simulink model "mdl5"  (R2014a)
settings: Solver=FixedStepDiscrete  SolverMode=SingleTasking  StartTime=TIME(1)  StopTime=TIME(end)  FixedStep=SIMSTEP  RelTol=1e-3
model workspace (MAT data in the model file):
  autoc_mdd_data01 : struct (value not decoded)
values from neighbouring files (symbols this model uses):
  map_mr4_01 = [400 500 600 700 800 900 1000 1100 1200 1300 1400 1500 ... (47 elements, 1x47)]    [scr_simdata_all.mat]
  map_mr4_02 = [0.684 0.622 0.566 0.514 0.468 0.425 0.387 0.352 0.32 0.291 0.264 0.241 ... (47 elements, 1x47)]    [scr_simdata_all.mat]
  map_mr4_03 = [10 12 14 16 18 20 22 24 26 28 30 32 ... (51 elements, 1x51)]    [scr_simdata_all.mat]
  map_mr4_04 = [0.0257 0.0124 0.00595 0.00286 0.00137 0.000662 0.000318 0.000153 7.37e-05 3.54e-05 1.7e-05 8.19e-06 ... (51 elements, 1x51)]    [scr_simdata_all.mat]
  map_mr4_05 = [10 12 14 16 18 20 22 24 26 28 30 32 ... (51 elements, 1x51)]    [scr_simdata_all.mat]
  map_mr4_06 = [0.9647 0.9835 0.9945 0.9994 0.9972 0.9871 0.97 0.9462 0.9163 0.8807 0.8403 0.796 ... (51 elements, 1x51)]    [scr_simdata_all.mat]
  map_mr4_07 = [0 1 2 3 4 5 6 7 8 9 10 11 ... (51 elements, 1x51)]    [scr_simdata_all.mat]
  map_mr4_08 = [0 0.01 0.0214 0.0335 0.0459 0.0587 0.0718 0.085 0.0985 0.112 0.126 0.14 ... (51 elements, 1x51)]    [scr_simdata_all.mat]
  Parameter114 = 126    [scr_simdata_all.mat]
  Parameter115 = 129    [scr_simdata_all.mat]
  Parameter131 = 3    [scr_simdata_all.mat]
  Parameter141 = 0    [scr_simdata_all.mat]
  Parameter143 = 1    [scr_simdata_all.mat]
  Parameter144 = 3    [scr_simdata_all.mat]
  Parameter51 = 0    [scr_simdata_all.mat]
  Parameter52 = 1    [scr_simdata_all.mat]
  Parameter53 = 2    [scr_simdata_all.mat]
  Parameter70 = 30    [scr_simdata_all.mat]
  Parameter71 = 33    [scr_simdata_all.mat]
  Parameter92 = 78    [scr_simdata_all.mat]
  Parameter93 = 81    [scr_simdata_all.mat]
  SIMSTEP = 0.0001024    [scr_simdata_all.mat]
(part 4 of 4)

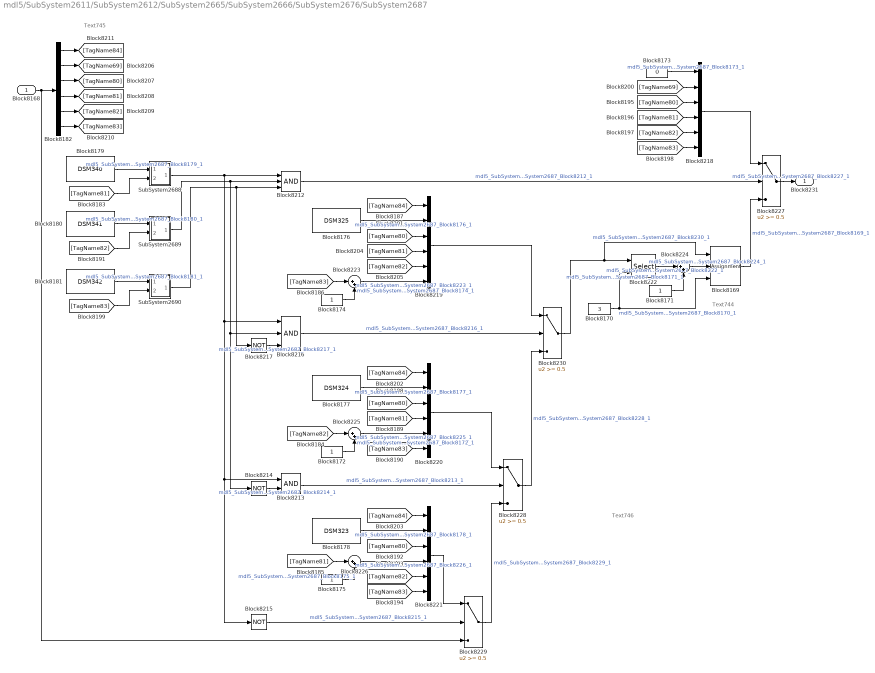
== system mdl5/SubSystem2611/SubSystem2612/SubSystem2665/SubSystem2666/SubSystem2676/SubSystem2687 ==
  note: Text746
  note: Text745
  note: Text744
  Block8168 : Inport
  Block8169 : Assignment  IndexOptions=Index vector (port)  OutputSizes=[1 1]
  Block8170 : Constant  Value=3  OutDataTypeStr=double  SampleTime=-1
  Block{8171..8172,8174..8175} (4 alike) : Constant  OutDataTypeStr=double  SampleTime=-1
  Block8173 : Constant  Value=0  OutDataTypeStr=double  SampleTime=-1
  Block8176 : DataStoreRead  DataStoreName=DSM325
  Block8177 : DataStoreRead  DataStoreName=DSM324
  Block8178 : DataStoreRead  DataStoreName=DSM323
  Block8179 : DataStoreRead  DataStoreName=DSM340
  Block8180 : DataStoreRead  DataStoreName=DSM341
  Block8181 : DataStoreRead  DataStoreName=DSM342
  Block8182 : Demux  Outputs=6
  Block8212 : Logic  Inputs=3
  Block8213 : Logic
  Block8214 : Logic  Operator=NOT
  Block8215 : Logic  Operator=NOT
  Block8216 : Logic  Inputs=3
  Block8217 : Logic  Operator=NOT
  Block{8218..8221} (4 alike) : Mux  Inputs=6
  Block8222 : Selector  IndexOptions=Index vector (port)  Indices=[1 3]
  Block{8223..8226} (4 alike) : Sum  Inputs=|++  OutDataTypeStr=double  RndMeth=Zero  SaturateOnIntegerOverflow=on  InputSameDT=on
  Block{8227..8230} (4 alike) : Switch  Threshold=0.5  RndMeth=Zero  SaturateOnIntegerOverflow=on  InputSameDT=on
  SubSystem2688 : Subsystem
  SubSystem2689 : Subsystem
  SubSystem2690 : Subsystem
  Block8231 : Outport
  wires:
  SubSystem2688/1(Out1) -> Block8212/1, Block8216/1, Block8213/1, Block8215/1
  SubSystem2689/1(Out1) -> Block8212/2, Block8216/2, Block8214/1
  SubSystem2690/1(Out1) -> Block8212/3, Block8217/1
  Block8212/1 -> Block8227/2  "mdl5_SubSystem2611_SubSystem2612_SubSystem2665_SubSystem2666_SubSystem2676_SubSystem2687_Block8212_1"
  Block8213/1 -> Block8228/2  "mdl5_SubSystem2611_SubSystem2612_SubSystem2665_SubSystem2666_SubSystem2676_SubSystem2687_Block8213_1"
  Block8215/1 -> Block8229/2  "mdl5_SubSystem2611_SubSystem2612_SubSystem2665_SubSystem2666_SubSystem2676_SubSystem2687_Block8215_1"
  Block8218/1 -> Block8227/1
  Block8179/1 -> SubSystem2688/1(In1)  "mdl5_SubSystem2611_SubSystem2612_SubSystem2665_SubSystem2666_SubSystem2676_SubSystem2687_Block8179_1"
  Block8180/1 -> SubSystem2689/1(In1)  "mdl5_SubSystem2611_SubSystem2612_SubSystem2665_SubSystem2666_SubSystem2676_SubSystem2687_Block8180_1"
  Block8181/1 -> SubSystem2690/1(In1)  "mdl5_SubSystem2611_SubSystem2612_SubSystem2665_SubSystem2666_SubSystem2676_SubSystem2687_Block8181_1"
  [TagName81] -> SubSystem2688/2(In2)
  [TagName82] -> SubSystem2689/2(In2)
  [TagName83] -> SubSystem2690/2(In2)
  Block8216/1 -> Block8230/2  "mdl5_SubSystem2611_SubSystem2612_SubSystem2665_SubSystem2666_SubSystem2676_SubSystem2687_Block8216_1"
  Block8219/1 -> Block8230/1
  Block8220/1 -> Block8228/1
  Block8221/1 -> Block8229/1
  Block8228/1 -> Block8230/3  "mdl5_SubSystem2611_SubSystem2612_SubSystem2665_SubSystem2666_SubSystem2676_SubSystem2687_Block8228_1"
  Block8229/1 -> Block8228/3  "mdl5_SubSystem2611_SubSystem2612_SubSystem2665_SubSystem2666_SubSystem2676_SubSystem2687_Block8229_1"
  Block8217/1 -> Block8216/3  "mdl5_SubSystem2611_SubSystem2612_SubSystem2665_SubSystem2666_SubSystem2676_SubSystem2687_Block8217_1"
  Block8214/1 -> Block8213/2  "mdl5_SubSystem2611_SubSystem2612_SubSystem2665_SubSystem2666_SubSystem2676_SubSystem2687_Block8214_1"
  Block8227/1 -> Block8231/1  "mdl5_SubSystem2611_SubSystem2612_SubSystem2665_SubSystem2666_SubSystem2676_SubSystem2687_Block8227_1"
  Block8173/1 -> Block8218/1  "mdl5_SubSystem2611_SubSystem2612_SubSystem2665_SubSystem2666_SubSystem2676_SubSystem2687_Block8173_1"
  [TagName69] -> Block8218/2
  [TagName80] -> Block8218/3
  [TagName81] -> Block8218/4
  [TagName82] -> Block8218/5
  [TagName83] -> Block8218/6
  [TagName84] -> Block8219/1
  [TagName80] -> Block8219/3
  [TagName81] -> Block8219/4
  [TagName82] -> Block8219/5
  Block8174/1 -> Block8223/2  "mdl5_SubSystem2611_SubSystem2612_SubSystem2665_SubSystem2666_SubSystem2676_SubSystem2687_Block8174_1"
  Block8176/1 -> Block8219/2  "mdl5_SubSystem2611_SubSystem2612_SubSystem2665_SubSystem2666_SubSystem2676_SubSystem2687_Block8176_1"
  Block8223/1 -> Block8219/6  "mdl5_SubSystem2611_SubSystem2612_SubSystem2665_SubSystem2666_SubSystem2676_SubSystem2687_Block8223_1"
  [TagName83] -> Block8223/1
  Block8169/1 -> Block8227/3  "mdl5_SubSystem2611_SubSystem2612_SubSystem2665_SubSystem2666_SubSystem2676_SubSystem2687_Block8169_1"
  Block8171/1 -> Block8224/2  "mdl5_SubSystem2611_SubSystem2612_SubSystem2665_SubSystem2666_SubSystem2676_SubSystem2687_Block8171_1"
  Block8224/1 -> Block8169/2  "mdl5_SubSystem2611_SubSystem2612_SubSystem2665_SubSystem2666_SubSystem2676_SubSystem2687_Block8224_1"
  Block8222/1 -> Block8224/1  "mdl5_SubSystem2611_SubSystem2612_SubSystem2665_SubSystem2666_SubSystem2676_SubSystem2687_Block8222_1"
  Block8170/1 -> Block8169/3, Block8222/2  "mdl5_SubSystem2611_SubSystem2612_SubSystem2665_SubSystem2666_SubSystem2676_SubSystem2687_Block8170_1"
  Block8230/1 -> Block8222/1, Block8169/1  "mdl5_SubSystem2611_SubSystem2612_SubSystem2665_SubSystem2666_SubSystem2676_SubSystem2687_Block8230_1"
  [TagName84] -> Block8220/1
  [TagName80] -> Block8220/3
  [TagName81] -> Block8220/4
  Block8225/1 -> Block8220/5  "mdl5_SubSystem2611_SubSystem2612_SubSystem2665_SubSystem2666_SubSystem2676_SubSystem2687_Block8225_1"
  Block8172/1 -> Block8225/2  "mdl5_SubSystem2611_SubSystem2612_SubSystem2665_SubSystem2666_SubSystem2676_SubSystem2687_Block8172_1"
  Block8177/1 -> Block8220/2  "mdl5_SubSystem2611_SubSystem2612_SubSystem2665_SubSystem2666_SubSystem2676_SubSystem2687_Block8177_1"
  [TagName83] -> Block8220/6
  [TagName82] -> Block8225/1
  [TagName84] -> Block8221/1
  [TagName80] -> Block8221/3
  Block8178/1 -> Block8221/2  "mdl5_SubSystem2611_SubSystem2612_SubSystem2665_SubSystem2666_SubSystem2676_SubSystem2687_Block8178_1"
  [TagName83] -> Block8221/6
  [TagName82] -> Block8221/5
  Block8226/1 -> Block8221/4  "mdl5_SubSystem2611_SubSystem2612_SubSystem2665_SubSystem2666_SubSystem2676_SubSystem2687_Block8226_1"
  Block8175/1 -> Block8226/2  "mdl5_SubSystem2611_SubSystem2612_SubSystem2665_SubSystem2666_SubSystem2676_SubSystem2687_Block8175_1"
  [TagName81] -> Block8226/1
  Block8182/1 -> [TagName84]
  Block8182/2 -> [TagName69]
  Block8182/3 -> [TagName80]
  Block8182/4 -> [TagName81]
  Block8182/5 -> [TagName82]
  Block8182/6 -> [TagName83]
  Block8168/1 -> Block8182/1, Block8229/3

== system mdl5/SubSystem2611/SubSystem2612/SubSystem2665/SubSystem2666/SubSystem2676/SubSystem2687/SubSystem2688 ==
  note: ***編集禁止***
  In1 : Inport
  In2 : Inport  Port=2
  RO1 : RelationalOperator  Operator===  InputSameDT=on
  single1 : DataTypeConversion  OutDataTypeStr=single  SaturateOnIntegerOverflow=on  RndMeth=Zero
  single2 : DataTypeConversion  OutDataTypeStr=single  SaturateOnIntegerOverflow=on  RndMeth=Zero
  Out1 : Outport
  wires:
  RO1/1 -> Out1/1  "mdl5_SubSystem2611_SubSystem2612_SubSystem2665_SubSystem2666_SubSystem2676_SubSystem2687_SubSystem2688_RO1_1"
  In2/1 -> single2/1
  In1/1 -> single1/1
  single1/1 -> RO1/1  "mdl5_SubSystem2611_SubSystem2612_SubSystem2665_SubSystem2666_SubSystem2676_SubSystem2687_SubSystem2688_single1_1"
  single2/1 -> RO1/2  "mdl5_SubSystem2611_SubSystem2612_SubSystem2665_SubSystem2666_SubSystem2676_SubSystem2687_SubSystem2688_single2_1"

== system mdl5/SubSystem2611/SubSystem2612/SubSystem2665/SubSystem2666/SubSystem2676/SubSystem2687/SubSystem2689 ==
  note: ***編集禁止***
  In1 : Inport
  In2 : Inport  Port=2
  RO1 : RelationalOperator  Operator===  InputSameDT=on
  single1 : DataTypeConversion  OutDataTypeStr=single  SaturateOnIntegerOverflow=on  RndMeth=Zero
  single2 : DataTypeConversion  OutDataTypeStr=single  SaturateOnIntegerOverflow=on  RndMeth=Zero
  Out1 : Outport
  wires:
  single2/1 -> RO1/2  "mdl5_SubSystem2611_SubSystem2612_SubSystem2665_SubSystem2666_SubSystem2676_SubSystem2687_SubSystem2689_single2_1"
  single1/1 -> RO1/1  "mdl5_SubSystem2611_SubSystem2612_SubSystem2665_SubSystem2666_SubSystem2676_SubSystem2687_SubSystem2689_single1_1"
  In1/1 -> single1/1
  In2/1 -> single2/1
  RO1/1 -> Out1/1  "mdl5_SubSystem2611_SubSystem2612_SubSystem2665_SubSystem2666_SubSystem2676_SubSystem2687_SubSystem2689_RO1_1"

== system mdl5/SubSystem2611/SubSystem2612/SubSystem2665/SubSystem2666/SubSystem2676/SubSystem2687/SubSystem2690 ==
  note: ***編集禁止***
  In1 : Inport
  In2 : Inport  Port=2
  RO1 : RelationalOperator  Operator===  InputSameDT=on
  single1 : DataTypeConversion  OutDataTypeStr=single  SaturateOnIntegerOverflow=on  RndMeth=Zero
  single2 : DataTypeConversion  OutDataTypeStr=single  SaturateOnIntegerOverflow=on  RndMeth=Zero
  Out1 : Outport
  wires:
  single2/1 -> RO1/2  "mdl5_SubSystem2611_SubSystem2612_SubSystem2665_SubSystem2666_SubSystem2676_SubSystem2687_SubSystem2690_single2_1"
  single1/1 -> RO1/1  "mdl5_SubSystem2611_SubSystem2612_SubSystem2665_SubSystem2666_SubSystem2676_SubSystem2687_SubSystem2690_single1_1"
  In1/1 -> single1/1
  In2/1 -> single2/1
  RO1/1 -> Out1/1  "mdl5_SubSystem2611_SubSystem2612_SubSystem2665_SubSystem2666_SubSystem2676_SubSystem2687_SubSystem2690_RO1_1"

== stateflow chart mdl5/SubSystem2611/SubSystem2691/SubSystem2693/SubSystem2694/For_loop ==
  note: for(i1 = 0; i1 < N_Loop; i1++) {
      |   処理
      | }
  (default) -> (junction 8) : {
      |  idx = 1;
      |  i1 = 0;
      | }
  (junction 11) -> (junction 8) : {i1++;}
  (junction 8) -> (junction 9)
  (junction 10) -> (junction 11) : {
      |  function_call;
      |  idx = idx + 1;
      | }
  (junction 9) -> (junction 10) [order 1] : [i1 < N_Loop]
  (junction 9) -> (junction 12) [order 2]
  data: N_Loop input; i1 local int32; idx output
  events: function_call output FUNCTION_CALL_EVENT
